simulink model "pd_control"  (R2022a)
settings: Solver=ode4  StartTime=0.0  StopTime=10.0  FixedStep=0.01  RelTol=1e-3
values from neighbouring files (symbols this model uses):
  den = [1  N]    [PD_only.m]    (also in PI_only.m = [1 0])
  Kd = K(i)    [PD_control_script.m]    (also in PD_only.m = 5)
  Kp = 1    [PD_control_script.m]    (also in PD_only.m; PI_only.m; Pi_control_script.m; p_control_script.m = K(i))
  N = 100    [PD_control_script.m]    (also in PD_only.m = Ni(i))
  num = [Kp+Kd*N  Kp*N]    [PD_control_script.m]    (also in PD_only.m = [Kp+Kd*N N]; PI_only.m = [Kp  Ki]; Pi_control_script.m = [Kp Ki]; i_control_script.m = Ki)
settings Model: Creator=김응태  LastModifiedBy=김응태

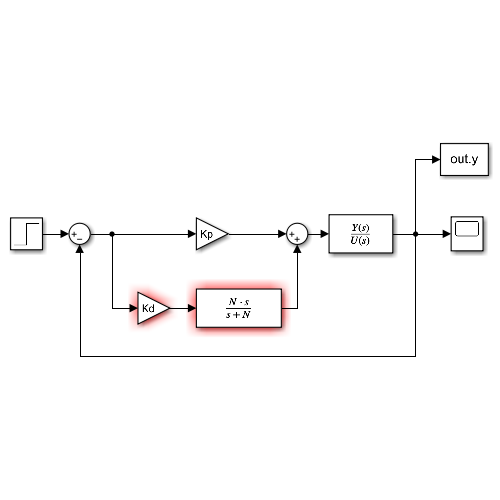
[thumbnail: Simulink's stored preview of the top-level diagram]
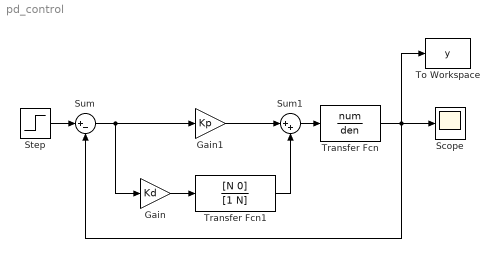
== system pd_control ==
  Gain : Gain  Gain=Kd
  Gain1 : Gain  Gain=Kp
  Scope : Scope
  Step : Step  Time=2  SampleTime=0
  Sum : Sum  Inputs=|+-
  Sum1 : Sum  Inputs=|++
  To Workspace : ToWorkspace  VariableName=y  SaveFormat=Timeseries  SampleTime=-1
  Transfer Fcn : TransferFcn  Numerator=num  Denominator=den
  Transfer Fcn1 : TransferFcn  Numerator=[N 0]  Denominator=[1 N]
  wires:
  Gain/1 -> Transfer Fcn1/1
  Step/1 -> Sum/1
  Transfer Fcn/1 -> Sum/2, To Workspace/1, Scope/1
  Sum1/1 -> Transfer Fcn/1
  Gain1/1 -> Sum1/1
  Transfer Fcn1/1 -> Sum1/2
  Sum/1 -> Gain/1, Gain1/1
